simulink model "FCElectricPlant"  (R2025b)
settings: Solver=VariableStepAuto  StartTime=0.0  StopTime=2474  RelTol=1e-3
model workspace (MAT data in the model file):
  Bat.DischrgLmt_bpt = [0 0.35 0.7 1 1 1 1 1 1 1 1]
  Bat.ChrgLmt_bpt = [1 1 1 1 1 1 1 1 0.7 0.35 0]
  Bat.SOC_bpt = [0 0.1 0.2 0.3 0.4 0.5 0.6 0.7 0.8 0.9 1]
  Bat.BattDischrgMax = 110000
  Bat.BattChrgMax = -110000
  Bat.noLoadV = [201.6  201.6  201.6  201.6  201.6  201.6  201.6; 258.768  258.768  258.768  258.768  258.768  258.768  258.768; 264.96  264.96  264.96  264.96  264.96  264.96  264.96; 272.952  272.952  272.952  272.952  272.952  272.952  272.952; 286.128  286.128  286.128  286.128  286.128  286.128  286.128; 303.912  303.912  303.912  303.912  303.912  303.912  303.912]
  Bat.CapSOCBp = [0 0.2 0.4 0.6 0.8 1]
  Bat.BattTempBp = [243.1 253.1 263.1 273.1 283.1 298.1 313.1]
  Bat.CapLUTBp = [0 0.01 0.02 0.03 0.04 0.05 0.06 0.07 0.08 0.09 0.1 0.11 0.12 0.13 0.14 0.15 0.16 0.17 0.18 0.19 0.2 0.21 0.22 0.23 0.24 0.25 0.26 0.27 0.28 0.29 0.3 0.31 0.32 0.33 0.34 0.35 0.36 0.37 0.38 0.39 0.4 0.41 0.42 0.43 0.44 0.45 0.46 0.47 0.48 0.49 0.5 0.51 0.52 0.53 0.54 0.55 0.56 0.57 0.58 0.59 0.6 0.61 0.62 0.63 0.64 0.65 0.66 0.67 0.68 0.69 0.7 0.71 0.72 0.73 0.74 0.75 0.76 0.77 0.78 0.79 0.8 0.81 0.82 0.83 0.84 0.85 0.86 0.87 0.88 0.89 0.9 0.91 0.92 0.93 0.94 0.95 0.96 0.97 0.98 0.99 1]
  Bat.Em = [2.8 3.228 3.284 3.361 3.408 3.427 3.472 3.477 3.493 3.504 3.516 3.528 3.537 3.545 3.555 3.561 3.566 3.576 3.587 3.589 3.594 3.6 3.608 3.61 3.616 3.619 3.626 3.632 3.637 3.64 3.645 3.646 3.652 3.655 3.658 3.661 3.664 3.668 3.673 3.678 3.68 3.681 3.686 3.692 3.699 3.702 3.705 3.71 3.717 3.723 3.728 3.733 3.735 3.742 3.749 3.755 3.761 3.768 3.773 3.78 3.791 3.798 3.798 3.814 3.818 3.825 3.841 3.846 3.855 3.863 3.877 3.885 3.894 3.907 3.919 3.926 3.935 3.944 3.954 3.964 3.974 3.988 3.998 4.014 4.029 4.034 4.047 4.065 4.074 4.086 4.097 4.131 4.126 4.138 4.15 4.18 4.174 4.187 4.207 4.231 4.221]
  Bat.Ns = 72
  Bat.Np = 2
  Bat.BattChargeMax = 5.3
  Bat.BattCapInit = 3.18
  Bat.AH = [5.3 5.3 5.3 5.3 5.3 5.3 5.3]
  Bat.initSOC = 0.6
  Bat.RInt = [0.008846  0.006389  0.004364  0.002031  0.001443  0.0005603  0.001028; 0.009319  0.006554  0.004101  0.002563  0.001825  0.0007192  0.001338; 0.009027  0.005553  0.00406  0.002532  0.001795  0.0006887  0.001; 0.00847  0.005525  0.003452  0.00246  0.001778  0.0007557  0.001536; 0.01032  0.006043  0.003846  0.002716  0.001924  0.0007355  0.001546; 0.01314  0.007805  0.004517  0.003047  0.002234  0.001014  0.002789]
  Bat.R0 = [0.636912  0.460008  0.314208  0.146232  0.103896  0.0403416  0.074016; 0.670968  0.471888  0.295272  0.184536  0.1314  0.0517824  0.096336; 0.649944  0.399816  0.29232  0.182304  0.12924  0.0495864  0.072; 0.60984  0.3978  0.248544  0.17712  0.128016  0.0544104  0.110592; 0.74304  0.435096  0.276912  0.195552  0.138528  0.052956  0.111312; 0.94608  0.56196  0.325224  0.219384  0.160848  0.073008  0.200808]
  Bat.thermalMass = 500
  BattDCDC.Vout = 650
  BattDCDC.Plim = 60000
  BattDCDC.currMax = 9230.76923077
  BattDCDC.eff = 98
  BattDCDC.convLoss = 1
  BattDCDC.tc = 0.001
  BattDCDC.Vinit = 650
  BattDCDC.thermalMass = 500
  BattDCDC.Vdroop = 0
  BattDCDC.avgSwitchResistance = 0.001
  BattDCDC.diodeFwdVolt = 0.8
  BattDCDC.diodeOnResistance = 0.001
  BattDCDC.diodeOffConductance = 1e-05
  BattDCDC.inductance = 0.005
  BattDCDC.inductorSeriesResistance = 0
  BattDCDC.capacitance = 0.001
  BattDCDC.CapEffSeriesResistance = 10
  Brk.BrkPrsMax = 5000000
  Brk.mu_kinetic = 0.35
  Brk.mu_static = 0.45
  Brk.disk_abore = 0.05
  Brk.Rm = 0.15
  Brk.num_pads = 2
  Cond.Width = 60
  Cond.Height = 40
  Cond.Thickness = 2
  Cond.Area = 2400
  Cond.TubeDh = 0.25
  Cond.TubeArea = 0.0490873852123
  Cond.NTube = 256
  Cond.NPerRow = 8
  Cond.NRows = 32
  Cond.Spacing = 1
  Cond.TotFinArea = 30720
  Cpl.GearRatio = 1
  Cpl.Friction = 0.0001
  DH2 = 74
  DH2O = 25
  DO2 = 18
  DRVctrl.Ki = 1
  DRVctrl.Kp = 2
  Diff.Ndiff = 7.94
  Diff.Inertia = 0.5
  Driveshaft.inertia = 3
  Duct.Length = 5
  Duct.Width = 60
  Duct.Height = 40
  Duct.Area = 2400
  Duct.Dh = 48
  ElecThermal.ctrl.Kp = 0.1
  ElecThermal.ctrl.Ki = 0.1
  ElecThermal.TM1.mass = 2
  ElecThermal.TM1.sh = 910
  ElecThermal.Tank.volume = 0.001
  ElecThermal.Tank.area = 0.005
  ElecThermal.Tank.heightVector = [0.01 0.01]
  ElecThermal.Tank.areaVectorA1B1 = [0.001 0.001]
  ElecThermal.Tank.areaVectorA2B2 = [7.85398163397e-05 7.85398163397e-05]
  ElecThermal.MassFlowSource.area = 7.85398163397e-05
  ElecThermal.TL.bulkMod = 2.1791
  ElecThermal.TL.PressMin = 0.01
  ElecThermal.TL.PressMax = 50
  ElecThermal.TL.volumeFraction = 0.1
  ElecThermal.LR1.area = 3.92699081699e-05
  ElecThermal.LR1.areaAB = 7.85398163397e-05
  ElecThermal.LR1.cd = 0.7
  ElecThermal.LR1.RN = 12
  ElecThermal.P1.length = 1
  ElecThermal.P1.area = 7.85398163397e-05
  ElecThermal.P1.diam = 0.01
  ElecThermal.P1.elevGain = 0
  ElecThermal.P1.eqLength = 0.1
  ElecThermal.P1.rough = 1.5e-05
  ElecThermal.P1.lamDarcyFrac = 64
  ElecThermal.P1.lamUpp = 2000
  ElecThermal.P1.turbLow = 4000
  ElecThermal.P1.lamNu = 3.66
  ElecThermal.P2.length = 1
  ElecThermal.P2.area = 7.85398163397e-05
  ElecThermal.P2.diam = 0.01
  ElecThermal.P2.elevGain = 0
  ElecThermal.P2.eqLength = 0.1
  ElecThermal.P2.rough = 1.5e-05
  ElecThermal.P2.lamDarcyFrac = 64
  ElecThermal.P2.lamUpp = 2000
  ElecThermal.P2.turbLow = 4000
  ElecThermal.P2.lamNu = 3.66
  ElecThermal.P3.length = 1
  ElecThermal.P3.area = 7.85398163397e-05
  ElecThermal.P3.diam = 0.01
  ElecThermal.P3.elevGain = 0
  ElecThermal.P3.eqLength = 0.1
  ElecThermal.P3.rough = 1.5e-05
  ElecThermal.P3.lamDarcyFrac = 64
  ElecThermal.P3.lamUpp = 2000
  ElecThermal.P3.turbLow = 4000
  ElecThermal.P3.lamNu = 3.66
  FCDCDC.Vout = 650
  FCDCDC.Plim = 60000
  FCDCDC.Vdroop = 0
  FCDCDC.currMax = 9230.76923077
  FCDCDC.eff = 98
  FCDCDC.convLoss = 1
  FCDCDC.tc = 0.001
  FCDCDC.Vinit = 650
  FCDCDC.thermalMass = 500
  FCDCDC.conductance = 1e-08
  FCDCDC.inductance = 0.005
  FCDCDC.capacitance = 0.001
  FCDCDC.diodeFwdVolt = 0.8
  FCDCDC.diodeOnResistance = 0.001
  FCDCDC.diodeOffConductance = 1e-05
  FCDCDC.avgSwitchResistance = 0.001
  FCDCDC.inductorSeriesResistance = 0
  FCDCDC.CapEffSeriesResistance = 10
  FCctrl.maxPWR = 128000
  FCctrl.opLimit = 0.4
  FCctrl.minV = 200
  FCctrl.SOCtgt = 60
  FCctrl.tempTgt = 80
  FTP72.time = [0 0.00166966283167 0.00489789127635 0.00812611972102 0.01 0.0132225488916 0.0164450977832 0.0196676466748 0.02 0.0216617666259 0.024481578167 0.0273013897082 ... (181869 elements, 181869x1)]
  FTP72.SpdKph = [0 0 0 0 0 0 0 0 0 0 0 0 ... (181869 elements, 181869x1)]
  FTP75.time = [0 0.00166966283167 0.00489789127635 0.00812611972102 0.01 0.0132225488916 0.0164450977832 0.0196676466748 0.02 0.0216617666259 0.024481578167 0.0273013897082 ... (325038 elements, 325038x1)]
  FTP75.SpdKph = [0 0 0 0 0 0 0 0 0 0 0 0 ... (325038 elements, 325038x1)]
  FinArea = 2
  FinDensity = 4
  H2_D = 74
  H2_R = 4124.48151676
  H2_T = [-56.55 -50 -40 -30 -20 -10 -5 -4 -3 -2 -1 0 1 2 3 4 5 10 20 30 40 50 60 70 80 90 100 110 120 130 140 150 160 170 180 190 200 210 220 230 240 250 260 270 280 290 300 310 320 330 340 350]
  H2_h = [2783.66044046 2873.94181646 3012.62601981 3152.22537302 3292.62486344 3433.7213836 3504.50184296 3518.67512521 3532.85394544 3547.03822323 3561.22787913 3575.42283463 3589.62301216 3603.82833507 3618.03872764 3632.25411507 3646.47442344 3717.6472553 3860.32198735 4003.38288163 4146.77354613 4290.44463594 4434.35318484 4578.46197843 4722.73896833 4867.15672726 5011.69194457 5156.32496144 5301.03934494 5445.82149962 5590.66031514 5735.54684833 5880.47403768 6025.43644827 6170.43004499 6315.451992 6460.50047605 6605.57455183 6750.67400705 6895.79924544 7040.95118569 7186.13117474 7331.34091359 7476.58239436 7621.85784699 7767.16969457 7912.52051596 8057.91301484 8203.34999414 8348.83433523 8494.36898091 8639.95692183]
  H2_k = [142.834673487 146.602208511 152.236222043 157.732550942 163.09765294 168.338595937 170.914793442 171.426608923 171.937300227 172.446874689 172.955339635 173.462702375 173.968970204 174.474150403 174.978250232 175.481276935 175.983237736 178.477304495 183.389581256 188.206454189 192.934525091 197.580042888 202.148890501 206.646585109 211.078287131 215.448814629 219.762660868 224.024013436 228.236773895 232.404577248 236.530810786 240.618632037 244.670985681 248.690619345 252.680098287 256.641818973 260.578021603 264.490801638 268.382120403 272.253814814 276.107606319 279.945109096 283.767837587 287.577213413 291.374571729 295.161167068 298.938178719 302.706715675 306.467821201 310.222477041 313.971607306 317.716082068]
  H2_mu = [7.13280985169 7.28192581803 7.50683010986 7.72860158312 7.94743907375 8.16352107178 8.27057966039 8.29191522386 8.31322574339 8.33451136221 8.35577222214 8.37700846366 8.39822022586 8.41940764654 8.44057086215 8.46171000786 8.48282521754 8.58804682376 8.79676834159 9.00329345223 9.20773222364 9.41018554309 9.61074613692 9.80949945112 10.0065244149 10.2018941058 10.3956763308 10.5879341365 10.7787262582 10.9681075163 11.1561291684 11.3428392212 11.5282827091 11.7125019432 11.8955367341 12.0774245926 12.2582009096 12.4378991192 12.6165508457 12.7941860372 12.9708330866 13.1465189421 13.3212692073 13.4951082332 13.668059202 13.8401442043 14.0113843094 14.1817996299 14.3514093822 14.5202319407 14.6882848893 14.8555850676]
  HWFET.time = [0 0.00166966283167 0.00489789127635 0.00812611972102 0.01 0.0132225488916 0.0164450977832 0.0196676466748 0.02 0.0216617666259 0.024481578167 0.0273013897082 ... (82069 elements, 82069x1)]
  HWFET.SpdKph = [0 0 0 0 0 0 0 0 0 0 0 0 ... (82069 elements, 82069x1)]
  Mot.maxT = [335 335 335 335 335 269.767628541 215.814102833 179.845085694 154.152930595 134.88381427 119.896723796 107.907051416]
  Mot.w_eff_bp = [0 1000 2000 3000 3221 4000 5000 6000 7000 8000 9000 10000]
  Mot.Tc_Mot = 0.02
  Mot.T_eff_bp = [0 23.9285714286 47.8571428571 71.7857142857 95.7142857143 119.642857143 143.571428571 167.5 191.428571429 215.357142857 239.285714286 263.214285714 287.142857143 311.071428571 335]
  Mot.efficiency_table = [85  85  85  85  85  85  85  85  85  85  85  85  85  85  85; 85  85  85  85  85  85  85  85  85  85  85  85  85  85  85; 85  85  90  90  90  90  90  90  90  90  88  88  88  88  88; 85  85  92  92  92  92  92  92  92  92  92  90  90  90  90; 85  85  92  92  93  93  93  93  92  92  92  90  90  90  90; 85  85  93  94  94  94  94  94  94  94  94  94  94  94  94; 85  85  93  94  94  95  95  95  95  95  95  95  95  95  95; 85  85  93  94  94  95  95  95  95  95  95  95  95  95  95; 85  85  93  94  95  95  95  95  95  95  95  95  95  95  95; 85  85  93  94  95  95  95  95  95  95  95  95  95  95  95; 85  85  93  94  94  94  94  94  94  94  94  94  94  94  94; 85  85  90  92  93  93  93  93  93  93  93  93  93  93  93]
  Mot.supplyRes = 0
  Mot.inertia = 5e-06
  Mot.damping = 0
  Mot.thermalMass = 800
  Mot.winding.area = 250.2
  Mot.winding.thick = 1
  Mot.winding.cond = 401
  Mot.winding.mass = 5
  Mot.winding.sh = 385
  Mot.windingIron.area = 250
  Mot.windingIron.thick = 1
  Mot.windingIron.cond = 360
  Mot.windingIron.mass = 5
  Mot.windingIron.sh = 447
  Mot.ironStack.area = 4350
  Mot.ironStack.thick = 1
  Mot.ironStack.cond = 80.2
  Mot.ironStack.mass = 5
  Mot.ironStack.sh = 903
  N2_R = 296.802103844
  N2_T = [-56.55 -50 -40 -30 -20 -10 -5 -4 -3 -2 -1 0 1 2 3 4 5 10 20 30 40 50 60 70 80 90 100 110 120 130 140 150 160 170 180 190 200 210 220 230 240 250 260 270 280 290 300 310 320 330 340 350]
  N2_h = [224.312019476 231.141016529 241.564116975 251.984329606 262.402210767 272.818266127 278.025759131 279.06722248 280.10867517 281.150117667 282.191550441 283.232973957 284.274388686 285.315795097 286.357193658 287.39858484 288.439969116 293.646803475 304.060229226 314.473742204 324.887858161 335.303123494 345.720119003 356.139461811 366.561805672 376.987839946 387.41828743 397.853901301 408.295461341 418.743769659 429.199646055 439.663923199 450.137441735 460.621045431 471.115576471 481.621870952 492.140754651 502.673039103 513.219518026 523.780964099 534.358126107 544.951726469 555.562459109 566.190987693 576.837944198 587.503927793 598.18950402 608.895204248 619.621525378 630.368929765 641.137845362 651.928666026]
  N2_k = [19.6296532607 20.1533289725 20.9436243616 21.7231523445 22.4923063139 23.2514823267 23.6274403303 23.7023472872 23.7771601873 23.8518793809 23.9265052168 24.0010380424 24.0754782033 24.1498260439 24.2240819071 24.298246134 24.3723190645 24.7413260601 25.4726839899 26.1954347636 26.9098870601 27.616335804 28.3150627088 29.0063368423 29.6904152006 30.3675432786 31.0379556302 31.7018764132 32.3595199136 33.0110910506 33.656785857 34.2967919383 34.9312889073 35.560448797 36.1844364511 36.8034098926 37.4175206728 38.0269141997 38.6317300489 39.2321022558 39.8281595918 40.4200258249 41.0078199644 41.591656493 42.1716455849 42.7478933118 43.3205018374 43.8895696009 44.4551914905 45.0174590069 45.5764604183 46.1322809066]
  N2_mu = [13.7948920665 14.1367187352 14.6513506072 15.1575394446 15.6556177861 16.1459023391 16.3882166949 16.4364580271 16.4846261831 16.532721447 16.5807441017 16.6286944287 16.6765727079 16.7243792177 16.7721142355 16.8197780369 16.8673708962 17.1042805671 17.572933093 18.0349108462 18.4904598525 18.9398140034 19.38319572 19.820816593 20.2528779961 20.6795716689 21.1010802692 21.5175778944 21.9292305719 22.3361967211 22.7386275856 23.1366676392 23.5304549666 23.9201216192 24.3057939489 24.6875929203 25.0656344035 25.4400294479 25.8108845388 26.1783018382 26.5423794103 26.9032114332 27.260888397 27.615497291 27.9671217779 28.3158423592 28.6617365294 29.0048789219 29.3453414462 29.6831934166 30.0185016744 30.3513307024]
  NFin = 7680
  O2_D = 18
  O2_R = 259.836612623
  O2_T = [-56.55 -50 -40 -30 -20 -10 -5 -4 -3 -2 -1 0 1 2 3 4 5 10 20 30 40 50 60 70 80 90 100 110 120 130 140 150 160 170 180 190 200 210 220 230 240 250 260 270 280 290 300 310 320 330 340 350]
  O2_h = [196.314045635 202.302438243 211.445560194 220.590899229 229.740231593 238.895348953 243.475641264 244.39194743 245.308340402 246.224821996 247.14139403 248.05805832 248.974816681 249.891670932 250.808622886 251.725674358 252.642827164 257.230174605 266.413508633 275.609852765 284.820965751 294.048557918 303.294277513 312.559698674 321.846311316 331.155513044 340.488603076 349.846778084 359.231129801 368.642644209 378.082202098 387.550580811 397.04845695 406.576409877 416.134925825 425.724402468 435.345153816 444.997415319 454.681349062 464.397049 474.144546127 483.92381355 493.734771414 503.577291639 513.451202454 523.356292707 533.292315938 543.258994208 553.256021689 563.283068012 573.339781379 583.425791441]
  O2_k = [19.6661951881 20.2224765128 21.0645207725 21.898029696 22.7232456338 23.5404090718 23.9460452976 24.0269406553 24.1077592592 24.1885013406 24.2691671302 24.349756858 24.4302707537 24.5107090462 24.5910719638 24.6713597344 24.751572585 25.1515209479 25.9459275198 26.7331962712 27.5135401678 28.2871691203 29.0542797087 29.8150645641 30.569709483 31.3183935589 32.0612893462 32.7985630479 33.5303747184 34.2568784759 34.9782227188 35.6945503443 36.4059989645 37.1127011203 37.81478449 38.5123720922 39.2055824827 39.8945299436 40.5793246667 41.2600729279 41.9368772562 42.6098365938 43.2790464498 43.9445990477 44.6065834647 45.2650857659 45.9201891311 46.5719739769 47.2205180715 47.8658966458 48.5081824976 49.1474460917]
  O2_mu = [15.7665575307 16.1727626079 16.7849249434 17.3877315055 17.9815180942 18.5666055809 18.8559834763 18.9136105725 18.9711555252 19.0286186248 19.0860001607 19.1433004205 19.2005196907 19.2576582565 19.3147164018 19.3716944089 19.4285925592 19.7118952085 20.2726692662 20.8258892364 21.3718096795 21.9106736607 22.4427133237 22.9681504449 23.4871969667 24.0000555078 24.5069198497 25.0079753989 25.5033996256 25.9933624783 26.4780267762 26.9575485797 27.4320775393 27.9017572254 28.3667254388 28.8271145028 29.2830515394 29.7346587283 30.1820535522 30.625349027 31.0646539191 31.5000729504 31.9317069915 32.3596532436 32.7840054112 33.2048538637 33.6222857893 34.0363853397 34.4472337669 34.8549095533 35.2594885333 35.6610440103]
  PTctrl.RegenBrkCutOff = [0 1]
  PTctrl.RegenBrkSpd_bpt = [5 9]
  Pipe.Length = 750
  Pipe.Dh = 1.5
  Pipe.Area = 1.76714586764
  Pump.Speed = 4000
  Pump.Displacement = 40
  RH2 = 4124.48291466
  RH2O = 461.523115726
  RH_a = 0.6
  RH_c = 0.6
  RN2 = 296.802204439
  RO2 = 259.836700689
  RelayVariant = 1
  ScenarioIndex = 5
  Sig = Simulink.Signal
  Sig.Dimensions = -1
  Sig.DimensionsMode = 'auto'
  Sig.Complexity = 'auto'
  Sig.SampleTime = -1
  Sig.SamplingMode = 'auto'
  Sig.DataType = 'auto'
  SimEndTime = 2474
  T_cell = 80
  T_eff_bp = [0 20 40 60 80 100 120 140 160 180 200 220 240 260 280]
  T_env = 20
  T_ext = 30
  T_init = 303.15
  Tank.Volume = 10
  Tank.Area = 625
  Tank.WallArea = 2850
  Tire.Inertia = 0.2
  Tire.Rated_Vertical_Load = 3000
  Tire.Rated_Peak_Long_Force = 3500
  Tire.Slip_At_Peak_Force = 6
  Tire.Radius = 0.3
  Tvec = [-50 -40 -30 -20 -10 0 10 20 30 40 50 60 70 80 90 100 110 120 130 140 150 160 170 180 190 200 210 220 230 240 250 260 270 280 290 300 310 320 330 340 350]
  US06.time = [0 0.00166966283167 0.00489789127635 0.00812611972102 0.01 0.0132225488916 0.0164450977832 0.0196676466748 0.02 0.0216617666259 0.024481578167 0.0273013897082 ... (72955 elements, 72955x1)]
  US06.SpdKph = [0 0 0 0 0 0 0 0 0 0 0 0 ... (72955 elements, 72955x1)]
  UrbanCycle1.time = [0; 1; 2; 3; 4; 5; 6; 7; 8; 9; 10; 11; 12; 13; 14; 15; 16; 17; 18; 19; 20; 21; 22; 23; 24; 25; 26; 27; 28; 29; 30; 31; 32; 33; 34; 35; 36; 37; 38; 39; 40; 41; 42; 43; 44; 45; 46; 47; 48; 49; 50; 51; 52; 53; 54; 55; 56; 57; 58; 59; 60; 61; 62; 63; 64; 65; 66; 67; 68; 69; 70; 71; 72; 73; 74; 75; 76; 77; 78; 79; 80; 81; 82; 83; 84; 85; 86; 87; 88; 89; 90; 91; 92; 93; 94; 95; 96; 97; 98; 99; 100; 101; 102; 103; 104; 105; 106; 107; 108; 109; 110; 111; 112; 113; 114; 115; 116; 117; 118; 119; 120; 121; 122; 123; 124; 125; 126; 127; 128; 129; 130; 131; 132; 133; 134; 135; 136; 137; 138; 139; 140; 141; 142; 143; 144; 145; 146; 147; 148; 149; 150; 151; 152; 153; 154; 155; 156; 157; 158; 159; 160; 161; 162; 163; 164; 165; 166; 167; 168; 169; 170; 171; 172; 173; 174; 175; 176; 177; 178; 179; 180; 181; 182; 183; 184; 185; 186; 187; 188; 189; 190; 191; 192; 193; 194; 195]
  UrbanCycle1.SpdKph = [0; 0; 0; 0; 0; 0; 0; 0; 0; 0; 0; 0; 3.8; 7.5; 11.3; 15; 15; 15; 15; 15; 15; 15; 15; 15; 12; 9; 6; 3; 0; 0; 0; 0; 0; 0; 0; 0; 0; 0; 0; 0; 0; 0; 0; 0; 0; 0; 0; 0; 0; 0; 2.7; 5.3; 8; 10.7; 13.3; 16; 18.7; 21.3; 24; 26.7; 29.3; 32; 32; 32; 32; 32; 32; 32; 32; 32; 32; 32; 32; 32; 32; 32; 32; 32; 32; 32; 32; 32; 32; 32; 32; 32; 29.1; 26.2; 23.3; 20.4; 17.5; 14.5; 11.6; 8.7; 5.8; 2.9; 0; 0; 0; 0; 0; 0; 0; 0; 0; 0; 0; 0; 0; 0; 0; 0; 0; 0; 0; 0; 0; 0; 1.9; 3.8; 5.8; 7.7; 9.6; 11.5; 13.5; 15.4; 17.3; 19.2; 21.2; 23.4; 25; 26.9; 28.8; 30.8; 32.7; 34.6; 36.5; 38.5; 40.4; 42.3; 44.2; 46.2; 48.1; 50; 50; 50; 50; 50; 50; 50; 50; 50; 50; 50; 50; 50; 48.1; 46.2; 44.4; 42.5; 40.6; 38.8; 36.9; 35; 35; 35; 35; 35; 35; 35; 35; 35; 35; 35; 35; 35; 35; 32.1; 29.2; 26.2; 23.3; 20.4; 17.5; 14.6; 11.7; 8.7; 5.8; 2.9; 0; 0; 0; 0; 0; 0; 0; 0]
  UrbanCycle2.SpdKph = [0; 0; 0; 0; 0; 0; 0; 0; 0; 0; 0; 0; 0; 0; 0; 0; 0; 0; 0; 0; 0; 3; 6; 9; 12; 15; 15; 15; 17.2; 19.4; 21.7; 23.9; 26.1; 28.3; 30.6; 32.8; 35; 35; 35; 36.9; 38.8; 40.6; 42.5; 44.4; 46.3; 48.1; 50; 50; 50; 51.5; 53.1; 54.6; 56.2; 57.7; 59.2; 60.8; 62.3; 63.8; 65.4; 66.9; 68.5; 70; 70; 70; 70; 70; 70; 70; 70; 70; 70; 70; 70; 70; 70; 70; 70; 70; 70; 70; 70; 70; 70; 70; 70; 70; 70; 70; 70; 70; 70; 70; 70; 70; 70; 70; 70; 70; 70; 70; 70; 70; 70; 70; 70; 70; 70; 70; 70; 70; 70; 70; 67.5; 65; 62.5; 60; 57.5; 55; 52.5; 50; 50; 50; 50; 50; 50; 50; 50; 50; 50; 50; 50; 50; 50; 50; 50; 50; 50; 50; 50; 50; 50; 50; 50; 50; 50; 50; 50; 50; 50; 50; 50; 50; 50; 50; 50; 50; 50; 50; 50; 50; 50; 50; 50; 50; 50; 50; 50; 50; 50; 50; 50; 50; 50; 50; 50; 50; 50; 50; 50; 50; 50; 50; 50; 50; 50; 50; 50; 50; 50; 51.5; 53.1; 54.6; 56.2; 57.7; 59.2; 60.8; 62.3; 63.8; 65.4; 66.9; 68.5; 70; 70; 70; 70; 70; 70; 70; 70; 70; 70; 70; 70; 70; 70; 70; 70; 70; 70; 70; 70; 70; 70; 70; 70; 70; 70; 70; 70; 70; 70; 70; 70; 70; 70; 70; 70; 70; 70; 70; 70; 70; 70; 70; 70; 70; 70; 70; 70; 70; 70; 70; 70.9; 71.7; 72.6; 73.4; 74.3; 75.1; 76; 76.9; 77.7; 78.6; 79.4; 80.3; 81.1; 82; 82.9; 83.7; 84.6; 85.4; 86.3; 87.1; 88; 88.9; 89.7; 90.6; 91.4; 92.3; 93.1; 94; 94.9; 95.7; 96.6; 97.4; 98.3; 99.1; 100; 100; 100; 100; 100; 100; 100; 100; 100; 100; 100; 100; 100; 100; 100; 100; 100; 100; 100; 100; 100; 100; 100; 100; 100; 100; 100; 100; 100; 100; 100; 101; 102; 103; 104; 105; 106; 107; 108; 109; 110; 111; 112; 113; 114; 115; 116; 117; 118; 119; 120; 120; 120; 120; 120; 120; 120; 120; 120; 120; 120; 117.5; 115; 112.5; 110; 107.5; 105; 102.5; 100; 97.5; 95; 92.5; 90; 87.5; 85; 82.5; 80; 76.3; 72.5; 68.8; 65; 61.3; 57.5; 53.8; 50; 45; 40; 35; 30; 25; 20; 15; 10; 5; 0; 0; 0; 0; 0; 0; 0; 0; 0; 0; 0; 0; 0; 0; 0; 0; 0; 0; 0; 0; 0]
  UrbanCycle2.time = [0; 1; 2; 3; 4; 5; 6; 7; 8; 9; 10; 11; 12; 13; 14; 15; 16; 17; 18; 19; 20; 21; 22; 23; 24; 25; 26; 27; 28; 29; 30; 31; 32; 33; 34; 35; 36; 37; 38; 39; 40; 41; 42; 43; 44; 45; 46; 47; 48; 49; 50; 51; 52; 53; 54; 55; 56; 57; 58; 59; 60; 61; 62; 63; 64; 65; 66; 67; 68; 69; 70; 71; 72; 73; 74; 75; 76; 77; 78; 79; 80; 81; 82; 83; 84; 85; 86; 87; 88; 89; 90; 91; 92; 93; 94; 95; 96; 97; 98; 99; 100; 101; 102; 103; 104; 105; 106; 107; 108; 109; 110; 111; 112; 113; 114; 115; 116; 117; 118; 119; 120; 121; 122; 123; 124; 125; 126; 127; 128; 129; 130; 131; 132; 133; 134; 135; 136; 137; 138; 139; 140; 141; 142; 143; 144; 145; 146; 147; 148; 149; 150; 151; 152; 153; 154; 155; 156; 157; 158; 159; 160; 161; 162; 163; 164; 165; 166; 167; 168; 169; 170; 171; 172; 173; 174; 175; 176; 177; 178; 179; 180; 181; 182; 183; 184; 185; 186; 187; 188; 189; 190; 191; 192; 193; 194; 195; 196; 197; 198; 199; 200; 201; 202; 203; 204; 205; 206; 207; 208; 209; 210; 211; 212; 213; 214; 215; 216; 217; 218; 219; 220; 221; 222; 223; 224; 225; 226; 227; 228; 229; 230; 231; 232; 233; 234; 235; 236; 237; 238; 239; 240; 241; 242; 243; 244; 245; 246; 247; 248; 249; 250; 251; 252; 253; 254; 255; 256; 257; 258; 259; 260; 261; 262; 263; 264; 265; 266; 267; 268; 269; 270; 271; 272; 273; 274; 275; 276; 277; 278; 279; 280; 281; 282; 283; 284; 285; 286; 287; 288; 289; 290; 291; 292; 293; 294; 295; 296; 297; 298; 299; 300; 301; 302; 303; 304; 305; 306; 307; 308; 309; 310; 311; 312; 313; 314; 315; 316; 317; 318; 319; 320; 321; 322; 323; 324; 325; 326; 327; 328; 329; 330; 331; 332; 333; 334; 335; 336; 337; 338; 339; 340; 341; 342; 343; 344; 345; 346; 347; 348; 349; 350; 351; 352; 353; 354; 355; 356; 357; 358; 359; 360; 361; 362; 363; 364; 365; 366; 367; 368; 369; 370; 371; 372; 373; 374; 375; 376; 377; 378; 379; 380; 381; 382; 383; 384; 385; 386; 387; 388; 389; 390; 391; 392; 393; 394; 395; 396; 397; 398; 399; 400]
  UrbanCycle3.time = [0; 1; 2; 3; 4; 5; 6; 7; 8; 9; 10; 11; 12; 13; 14; 15; 16; 17; 18; 19; 20; 21; 22; 23; 24; 25; 26; 27; 28; 29; 30; 31; 32; 33; 34; 35; 36; 37; 38; 39; 40; 41; 42; 43; 44; 45; 46; 47; 48; 49; 50; 51; 52; 53; 54; 55; 56; 57; 58; 59; 60; 61; 62; 63; 64; 65; 66; 67; 68; 69; 70; 71; 72; 73; 74; 75; 76; 77; 78; 79; 80; 81; 82; 83; 84; 85; 86; 87; 88; 89; 90; 91; 92; 93; 94; 95; 96; 97; 98; 99; 100; 101; 102; 103; 104; 105; 106; 107; 108; 109; 110; 111; 112; 113; 114; 115; 116; 117; 118; 119; 120; 121; 122; 123; 124; 125; 126; 127; 128; 129; 130; 131; 132; 133; 134; 135; 136; 137; 138; 139; 140; 141; 142; 143; 144; 145; 146; 147; 148; 149; 150; 151; 152; 153; 154; 155; 156; 157; 158; 159; 160; 161; 162; 163; 164; 165; 166; 167; 168; 169; 170; 171; 172; 173; 174; 175; 176; 177; 178; 179; 180; 181; 182; 183; 184; 185; 186; 187; 188; 189; 190; 191; 192; 193; 194; 195; 196; 197; 198; 199; 200; 201; 202; 203; 204; 205; 206; 207; 208; 209; 210; 211; 212; 213; 214; 215; 216; 217; 218; 219; 220; 221; 222; 223; 224; 225; 226; 227; 228; 229; 230; 231; 232; 233; 234; 235; 236; 237; 238; 239; 240; 241; 242; 243; 244; 245; 246; 247; 248; 249; 250; 251; 252; 253; 254; 255; 256; 257; 258; 259; 260; 261; 262; 263; 264; 265; 266; 267; 268; 269; 270; 271; 272; 273; 274; 275; 276; 277; 278; 279; 280; 281; 282; 283; 284; 285; 286; 287; 288; 289; 290; 291; 292; 293; 294; 295; 296; 297; 298; 299; 300; 301; 302; 303; 304; 305; 306; 307; 308; 309; 310; 311; 312; 313; 314; 315; 316; 317; 318; 319; 320; 321; 322; 323; 324; 325; 326; 327; 328; 329; 330; 331; 332; 333; 334; 335; 336; 337; 338; 339; 340; 341; 342; 343; 344; 345; 346; 347; 348; 349; 350; 351; 352; 353; 354; 355; 356; 357; 358; 359; 360; 361; 362; 363; 364; 365; 366; 367; 368; 369; 370; 371; 372; 373; 374; 375; 376; 377; 378; 379; 380; 381; 382; 383; 384; 385; 386; 387; 388; 389; 390; 391; 392; 393; 394; 395; 396; 397; 398; 399; 400]
  UrbanCycle3.SpdKph = [0; 0; 0; 0; 0; 0; 0; 0; 0; 0; 0; 0; 0; 0; 0; 0; 0; 0; 0; 0; 0; 3; 6; 9; 12; 15; 15; 15; 17.2; 19.4; 21.7; 23.9; 26.1; 28.3; 30.6; 32.8; 35; 35; 35; 36.9; 38.8; 40.6; 42.5; 44.4; 46.3; 48.1; 50; 50; 50; 51.5; 53.1; 54.6; 56.2; 57.7; 59.2; 60.8; 62.3; 63.8; 65.4; 66.9; 68.5; 70; 70; 70; 70; 70; 70; 70; 70; 70; 70; 70; 70; 70; 70; 70; 70; 70; 70; 70; 70; 70; 70; 70; 70; 70; 70; 70; 70; 70; 70; 70; 70; 70; 70; 70; 70; 70; 70; 70; 70; 70; 70; 70; 70; 70; 70; 70; 70; 70; 70; 70; 67.5; 65; 62.5; 60; 57.5; 55; 52.5; 50; 50; 50; 50; 50; 50; 50; 50; 50; 50; 50; 50; 50; 50; 50; 50; 50; 50; 50; 50; 50; 50; 50; 50; 50; 50; 50; 50; 50; 50; 50; 50; 50; 50; 50; 50; 50; 50; 50; 50; 50; 50; 50; 50; 50; 50; 50; 50; 50; 50; 50; 50; 50; 50; 50; 50; 50; 50; 50; 50; 50; 50; 50; 50; 50; 50; 50; 50; 50; 50; 51.5; 53.1; 54.6; 56.2; 57.7; 59.2; 60.8; 62.3; 63.8; 65.4; 66.9; 68.5; 70; 70; 70; 70; 70; 70; 70; 70; 70; 70; 70; 70; 70; 70; 70; 70; 70; 70; 70; 70; 70; 70; 70; 70; 70; 70; 70; 70; 70; 70; 70; 70; 70; 70; 70; 70; 70; 70; 70; 70; 70; 70; 70; 70; 70; 70; 70; 70; 70; 70; 70; 70.8; 71.7; 72.5; 73.3; 74.2; 75; 75.8; 76.7; 77.5; 78.3; 79.2; 80; 80.8; 81.7; 82.5; 83.3; 84.2; 85; 85.8; 86.7; 87.5; 88.3; 89.2; 90; 90; 90; 90; 90; 90; 90; 90; 90; 90; 90; 90; 90; 90; 90; 90; 90; 90; 90; 90; 90; 90; 90; 90; 90; 90; 90; 90; 90; 90; 90; 90; 90; 90; 90; 90; 90; 90; 90; 90; 90; 90; 90; 90; 90; 90; 90; 90; 90; 90; 90; 90; 90; 90; 90; 90; 90; 90; 90; 90; 90; 90; 90; 90; 90; 90; 90; 90; 90; 90; 90; 90; 90; 90; 90; 90; 90; 90; 90; 90; 90; 90; 90; 90; 87.5; 85; 82.5; 80; 76.3; 72.5; 68.8; 65; 61.3; 57.5; 53.8; 50; 45; 40; 35; 30; 25; 20; 15; 10; 5; 0; 0; 0; 0; 0; 0; 0; 0; 0; 0; 0; 0; 0; 0; 0; 0; 0; 0; 0; 0; 0]
  UrbanCycle4.time = [0 1 2 3 4 5 6 7 8 9 10 11 ... (507 elements, 507x1)]
  UrbanCycle4.SpdKph = [0 0 0 0 0 0 0 0 0 0 0 0 ... (507 elements, 507x1)]
  UrbanCycle5.time = [0 1 2 3 4 5 6 7 8 9 10 11 ... (661 elements, 661x1)]
  UrbanCycle5.SpdKph = [0 0 0 0 0 0 0 0 0 0 0 0 ... (661 elements, 661x1)]
  Vehicle.Mass = 1800
  Vehicle.Distance_CG_FrontAxle = 1.35
  Vehicle.Distance_CG_RearAxle = 1.35
  Vehicle.Distance_CG_Ground = 0.5
  Vehicle.Frontal_Area = 2.16
  Vehicle.Aero_Drag_Coeff = 0.26
  WOT.time = [0 0.00166966283167 0.00489789127635 0.00812611972102 0.01 0.0132225488916 0.0164450977832 0.0196676466748 0.02 0.0216617666259 0.024481578167 0.0273013897082 ... (6347 elements, 6347x1)]
  WOT.SpdKph = [0 0 0 0 0 0 0 0 0 0 0 0 ... (6347 elements, 6347x1)]
  anode_tube_D = 0.01
  cathode_tube_D = 0.05
  comp_mdot_corr_TLU = [0  0.2  0.4; 0  0.15  0.3; 0  0.1  0.2; 0  0.05  0.1; 0  0  0]
  comp_p_ratio_TLU = [1; 1.25; 1.5; 1.75; 2]
  comp_rpm_TLU = [0 1800 3600]
  coolant_num_layers = 20
  coolant_num_passes = 12
  coolant_tube_D = 0.05
  coolant_w_channels = 1
  drive_cycle_power = [0 0 0 0 0 0 0 0 0 0 0 0 ... (1050 elements, 1050x1)]
  drive_cycle_time = [0 3.15544362088e-30 0.0046730644306 0.0046730644306 0.0229169980413 0.0229169980413 0.0411609316521 0.0594048652628 0.0958927324843 0.168868466927 0.308339923682 0.308339923682 ... (1050 elements, 1050x1)]
  efficiency_table = [85  85  85  85  85  85  85  85  85  85  85  85  85  85  85; 85  85  85  85  85  85  85  85  85  85  85  85  85  85  85; 85  85  90  90  90  90  90  90  90  90  88  88  88  88  88; 85  85  92  92  92  92  92  92  92  92  92  90  90  90  90; 85  85  92  92  93  93  93  93  92  92  92  90  90  90  90; 85  85  93  94  94  94  94  94  94  94  94  94  94  94  94; 85  85  93  94  94  95  95  95  95  95  95  95  95  95  95; 85  85  93  94  94  95  95  95  95  95  95  95  95  95  95; 85  85  93  94  95  95  95  95  95  95  95  95  95  95  95; 85  85  93  94  95  95  95  95  95  95  95  95  95  95  95; 85  85  93  94  94  94  94  94  94  94  94  94  94  94  94; 85  85  90  92  93  93  93  93  93  93  93  93  93  93  93]
  env_RH = 0.5
  env_T = 20
  env_p = 0.101325
  env_yO2 = 0.21
  f_fc_auxpower = [551.873653203 546.0853282 528.48462663 513.173595038 503.302975177 502.753456089 515.021163214 542.265022773 584.751680012 640.816461254 707.312051903 780.384247238 ... (869 elements, 79x11)]
  f_fc_currcmd_bpt = [0.209765 5.20060185897 10.1914387179 15.1822755769 20.1731124359 25.1639492949 30.1547861538 35.1456230128 40.1364598718 45.1272967308 50.1181335897 55.1089704487 60.0998073077 65.0906441667 70.0814810256 75.0723178846 80.0631547436 85.0539916026 90.0448284615 95.0356653205 100.026502179 105.017339038 110.008175897 114.999012756 119.989849615 124.980686474 129.971523333 134.962360192 139.953197051 144.94403391 149.934870769 154.925707628 159.916544487 164.907381346 169.898218205 174.889055064 179.879891923 184.870728782 189.861565641 194.8524025 199.843239359 204.834076218 209.824913077 214.815749936 219.806586795 224.797423654 229.788260513 234.779097372 239.769934231 244.76077109 249.751607949 254.742444808 259.733281667 264.724118526 269.714955385 274.705792244 279.696629103 284.687465962 289.678302821 294.669139679 299.659976538 304.650813397 309.641650256 314.632487115 319.623323974 324.614160833 329.604997692 334.595834551 339.58667141 344.577508269 349.568345128 354.559181987 359.550018846 364.540855705 369.531692564 374.522529423 379.513366282 384.504203141 389.49504]
  f_fc_h2flow = [8.71593619412e-08 2.11208831613e-05 4.21802637945e-05 6.3315607286e-05 8.44733435522e-05 0.000105614873893 0.000126714989157 0.000147760022647 0.000168745833381 0.000189675717181 0.000210558338983 0.000231405772833 ... (869 elements, 79x11)]
  f_fc_heatflow = [-113.508553924 315.682858012 683.83093304 1077.33211881 1492.74924564 1928.28255982 2383.1090309 2856.86201514 3349.28475785 3860.05320307 4388.73420272 4934.82889994 ... (869 elements, 79x11)]
  f_fc_tmpcmd_bpt = [50 55 60 65 70 75 80 85 90 95 100]
  f_fc_voltage = [454.992615106 449.926167951 444.44198715 439.413829244 434.829610174 430.668984057 426.90491616 423.505302786 420.434569606 417.655187333 415.129053553 412.818701247 ... (869 elements, 79x11)]
  hH2 = [2873941.81645 3012626.01981 3152225.37301 3292624.86344 3433721.38359 3575422.83463 3717647.2553 3860321.98734 4003382.88163 4146773.54613 4290444.63593 4434353.18483 4578461.97843 4722738.96833 4867156.72726 5011691.94456 5156324.96143 5301039.34494 5445821.49962 5590660.31514 5735546.84833 5880474.03768 6025436.44826 6170430.04499 6315451.99199 6460500.47604 6605574.55182 6750674.00704 6895799.24543 7040951.18568 7186131.17473 7331340.91359 7476582.39435 7621857.84698 7767169.69456 7912520.51596 8057913.01483 8203349.99414 8348834.33523 8494368.98091 8639956.92183]
  hH2O = [2407979.18389 2426599.35505 2445219.52621 2463839.69737 2482459.86853 2501080.03969 2520041.36444 2538661.5356 2557304.93352 2575974.09714 2594671.5511 2613399.77792 2632161.19415 2650958.13077 2669792.81764 2688667.37205 2707583.79088 2726543.94613 2745549.58335 2764602.32251 2783703.66092 2802854.97781 2822057.54008 2841312.50904 2860620.94768 2879983.8283 2899402.0402 2918876.39739 2938407.64597 2957996.47114 2977643.50384 2997349.32672 3017114.47952 3036939.46377 3056824.74662 3076770.76378 3096777.92136 3116846.59619 3136977.13407 3157169.84449 3177424.99]
  hN2 = [231141.016491 241564.116943 251984.329578 262402.210743 272818.266107 283232.973942 293646.803464 304060.22922 314473.742203 324887.858166 335303.123505 345720.119022 356139.461838 366561.80571 376987.839995 387418.287492 397853.901378 408295.461435 418743.769771 429199.646188 439663.923356 450137.441917 460621.045642 471115.576713 481621.871228 492140.754963 502673.039455 513219.518421 523780.964538 534358.126595 544951.727008 555562.459702 566190.988344 576837.944909 587503.928567 598189.50486 608895.205157 619621.526358 630368.93082 641137.846494 651928.667237]
  hO2 = [202302.438244 211445.560195 220590.89923 229740.231594 238895.348953 248058.05832 257230.174606 266413.508634 275609.852766 284820.965752 294048.557919 303294.277514 312559.698674 321846.311316 331155.513045 340488.603077 349846.778085 359231.129802 368642.644209 378082.202099 387550.580812 397048.456951 406576.409878 416134.925826 425724.402468 435345.153817 444997.41532 454681.349063 464397.049001 474144.546128 483923.813551 493734.771415 503577.291639 513451.202454 523356.292708 533292.315939 543258.994209 553256.02169 563283.068013 573339.78138 583425.791442]
  hvH2O = [2837864.0802 2838666.81899 2838713.54467 2838009.25742 2836579.406 2834477.18894 2477187.06302 2453519.25942 2429811.22988 2405977.28679 2381947.12654 2357654.5203 2333031.20801 2308003.52809 2282490.62772 2256403.72153 2229646.15315 2202114.07337 2173697.48076 2144281.28269 2113746.00965 2081967.88341 2048818.0713 2014161.09963 1977852.49331 1939735.72817 1899638.5239 1857368.38273 1812707.10332 1765403.78805 1715165.61416 1661645.2634 1604423.22494 1542982.06457 1476667.90089 1404630.83498 1325728.75296 1238362.12284 1140162.8135 1027316.58329 892746.804216]
  kH2 = [0.14660211438 0.15223611697 0.157732436203 0.163097529696 0.168338465237 0.173462565161 0.178477161614 0.183389433463 0.188206302164 0.192934369439 0.197579884152 0.202148729169 0.206646421619 0.211078121877 0.215448647967 0.21976249312 0.224023844894 0.228236604824 0.232404407893 0.236530641368 0.240618462761 0.244670816735 0.248690450904 0.252679930513 0.256641652017 0.260577855606 0.264490636733 0.268381956715 0.272253652461 0.276107445413 0.279944949744 0.283767679891 0.287577057471 0.291374417634 0.295161014911 0.298938028586 0.302706567652 0.30646767537 0.310222333482 0.313971466098 0.317715943287]
  kH2O = [0.0133993325489 0.0140727292017 0.0147461258545 0.0154195225073 0.0160929191601 0.0167663158129 0.017416450238 0.0180898468908 0.0187835182831 0.019496836926 0.0202291830642 0.0209799564979 0.0217485824984 0.022534514185 0.0233372328149 0.0241562468853 0.0249910906022 0.0258413220573 0.0267065213239 0.027586288594 0.0284802424289 0.0293880181591 0.0303092664468 0.0312436520137 0.0321908525251 0.0331505576189 0.0341224680656 0.0351062950429 0.0361017595124 0.0371085916839 0.0381265305554 0.039155323521 0.0401947260356 0.0412445013363 0.0423044202141 0.0433742608421 0.0444538086676 0.0455428563902 0.046641204073 0.047748659475 0.048865038743]
  kN2 = [0.0201533289599 0.0209436243479 0.0217231523299 0.0224923062983 0.0232514823103 0.0240010380251 0.0247413260421 0.0254726839711 0.026195434744 0.0269098870397 0.0276163357829 0.028315062687 0.0290063368199 0.0296904151774 0.0303675432547 0.0310379556057 0.031701876388 0.0323595198879 0.0330110910242 0.03365678583 0.0342967919107 0.0349312888791 0.0355604487682 0.0361844364218 0.0368034098627 0.0374175206423 0.0380269141687 0.0386317300173 0.0392321022236 0.0398281595592 0.0404200257917 0.0410078199307 0.0415916564588 0.0421716455502 0.0427478932766 0.0433205018017 0.0438895695647 0.0444551914538 0.0450174589697 0.0455764603806 0.0461322808684]
  kO2 = [0.0202224764979 0.0210645207571 0.0218980296803 0.0227232456176 0.0235404090551 0.0243497568408 0.0251515209302 0.0259459275017 0.0267331962527 0.0275135401488 0.0282871691008 0.0290542796888 0.0298150645436 0.0305697094621 0.0313183935376 0.0320612893244 0.0327985630256 0.0335303746957 0.0342568784527 0.0349782226953 0.0356945503203 0.03640599894 0.0371127010954 0.0378147844647 0.0385123720666 0.0392055824566 0.0398945299172 0.0405793246398 0.0412600729007 0.0419368772286 0.0426098365657 0.0432790464214 0.0439445990189 0.0446065834356 0.0452650857363 0.0459201891012 0.0465719739465 0.0472205180409 0.0478658966148 0.0485081824662 0.04914744606]
  muH2 = [7.28192631884e-06 7.50683062629e-06 7.72860211493e-06 7.94743962074e-06 8.16352163375e-06 8.37700904042e-06 8.58804741514e-06 8.79676894741e-06 9.00329407235e-06 9.20773285791e-06 9.41018619135e-06 9.61074679906e-06 9.809500127e-06 1.00065251044e-05 1.02018948088e-05 1.03956770472e-05 1.05879348662e-05 1.0778727001e-05 1.09681082723e-05 1.11561299374e-05 1.1342840003e-05 1.15282835037e-05 1.17125027505e-05 1.18955375541e-05 1.20774254252e-05 1.22582017546e-05 1.24378999766e-05 1.26165517154e-05 1.27941869192e-05 1.29708339808e-05 1.31465198485e-05 1.33212701257e-05 1.34951091636e-05 1.36680601444e-05 1.38401451585e-05 1.40113852754e-05 1.41818006077e-05 1.43514103717e-05 1.45202329419e-05 1.4688285902e-05 1.48555860919e-05]
  muH2O = [7.40754821278e-06 7.71570492949e-06 8.0238616462e-06 8.33201836291e-06 8.64017507962e-06 8.94833179633e-06 9.24231634895e-06 9.55047306566e-06 9.87031914628e-06 1.02003383346e-05 1.05392900589e-05 1.08861429187e-05 1.12400271296e-05 1.16001998721e-05 1.19660196026e-05 1.23369267066e-05 1.27124287135e-05 1.30920888432e-05 1.34755170214e-05 1.38623627459e-05 1.42523093607e-05 1.46450694092e-05 1.50403808272e-05 1.54380037934e-05 1.5837718101e-05 1.6239320946e-05 1.66426250507e-05 1.70474570612e-05 1.74536561678e-05 1.78610729109e-05 1.82695681407e-05 1.86790121055e-05 1.90892836493e-05 1.9500269501e-05 1.99118636434e-05 2.03239667489e-05 2.07364856747e-05 2.11493330075e-05 2.15624266528e-05 2.19756894601e-05 2.23890488821e-05]
  muN2 = [1.41367187228e-05 1.46513505944e-05 1.51575394313e-05 1.56556177724e-05 1.6145902325e-05 1.66286944141e-05 1.71042805521e-05 1.75729330776e-05 1.80349108304e-05 1.84904598363e-05 1.89398139868e-05 1.9383195703e-05 1.98208165756e-05 2.02528779784e-05 2.06795716508e-05 2.11010802507e-05 2.15175778755e-05 2.19292305527e-05 2.23361967016e-05 2.27386275656e-05 2.31366676189e-05 2.3530454946e-05 2.39201215982e-05 2.43057939276e-05 2.46875928987e-05 2.50656343816e-05 2.54400294256e-05 2.58108845161e-05 2.61783018152e-05 2.6542379387e-05 2.69032114096e-05 2.72608883731e-05 2.76154972668e-05 2.79671217534e-05 2.83158423343e-05 2.86617365042e-05 2.90048788965e-05 2.93453414205e-05 2.96831933906e-05 3.00185016481e-05 3.03513306758e-05]
  muO2 = [1.6172762594e-05 1.67849249289e-05 1.73877314906e-05 1.79815180788e-05 1.8566605565e-05 1.9143300404e-05 1.97118951916e-05 2.02726692488e-05 2.08258892185e-05 2.13718096611e-05 2.19106736419e-05 2.24427133044e-05 2.29681504252e-05 2.34871969465e-05 2.40000554872e-05 2.45069198286e-05 2.50079753774e-05 2.55033996037e-05 2.59933624559e-05 2.64780267534e-05 2.69575485565e-05 2.74320775157e-05 2.79017572014e-05 2.83667254144e-05 2.88271144781e-05 2.92830515142e-05 2.97346587027e-05 3.01820535262e-05 3.06253490007e-05 3.10646538924e-05 3.15000729233e-05 3.1931706964e-05 3.23596532158e-05 3.2784005383e-05 3.32048538352e-05 3.36222857604e-05 3.40363853104e-05 3.44472337373e-05 3.48549095233e-05 3.5259488503e-05 3.56610439797e-05]
  pH2O = [0.0039376926592 0.0128411282011 0.0380050105363 0.103238678713 0.259872929049 0.611151401419 1.22819893069 2.33931818334 4.24697083683 7.38493807375 12.3519458375 19.9464343078 31.2009300265 47.4144740302 70.1817658151 101.41799666 143.378712949 198.67442048 270.279976785 361.5390994 476.16453797 618.234621425 792.187006981 1002.81053608 1255.23615516 1554.92790047 1907.67499353 2319.5861702 2797.08749693 3346.92514427 3976.17493065 4692.2609923 5502.98678301 6416.58290953 7441.77834442 8587.90494083 9865.05121118 11284.2929275 12858.0516 14600.6773719 16529.415139]
  p_a = 0.101325
  p_c = 0.101325
  p_sat = 0.0474144740302
  p_sat_c = 0.0474144740302
  p_sat_e = 0.00233931818334
  radiator_H = 0.5
  radiator_L = 1
  radiator_N_fins = 12000
  radiator_N_tubes = 25
  radiator_W = 0.025
  radiator_air_area_fins = 11.5625
  radiator_air_area_primary = 1.223125
  radiator_cp = 910
  radiator_eta_fin = 0.7
  radiator_fin_spacing = 0.002
  radiator_gap_H = 0.0192708333333
  radiator_rho = 2700
  radiator_t_wall = 0.0001
  radiator_tube_H = 0.0015
  radiator_tube_Leq = 2.5
  stack_D_gdl = 0.07
  stack_alpha = 0.6
  stack_area = 280
  stack_iL = 1.4
  stack_io = 0.0001
  stack_mea_cp = 870
  stack_mea_rho = 1800
  stack_membrane_MW = 1.1
  stack_membrane_rho = 2000
  stack_num_cells = 400
  stack_num_channels = 8
  stack_t_gdl = 250
  stack_t_membrane = 125
  stack_w_channels = 1
  tank_V = 120
  tank_p = 70
  tank_yH2 = 0.9997
  y_H2O_a = 0.280766685597
  y_H2O_c = 0.0138523652603
  y_H2_a = 0.719233314403
  y_N2_a = 0
  y_N2_c = 0.77614763474
  y_O2_c = 0.21
libraries: fl_lib x91, nesl_utility x43, autolibpowerinfoutils x9, SimscapeFluids_lib x5, ee_lib x3, slpidlib x2, batteryecm_lib x1, simulink_extras x1, simulink x1
(part 1 of 4)
settings Model: DataDictionary=FCElectricPlant.sldd  ModifiedByFormat=The MathWorks, Inc.  SimulationMode=accelerator  Creator=The MathWorks, Inc.  LastModifiedBy=The MathWorks, Inc.
settings SolverCC: ZeroCrossAlgorithm=Adaptive  AlgebraicLoopSolver=TrustRegion  AutoInsertRateTranBlk=on  DecoupledContinuousIntegration=on  MinimalZcImpactIntegration=on  MaxZcPerStep=1.0
settings DataIOCC: SaveOutput=off  DSMLogging=off  SaveTime=off  ReturnWorkspaceOutputs=off
settings OptimizationCC: ReuseModelBlockBuffer=off  EfficientMapNaN2IntZero=off
settings DebuggingCC: ArtificialAlgebraicLoopMsg=none  MaskedZcDiagnostic=none  IgnoredZcDiagnostic=none  UnconnectedInputMsg=warning  UnconnectedOutputMsg=warning  UnconnectedLineMsg=warning  SubsystemReferenceDiagnosticForUnitTest=warning  SymbolicDimsDataTypeCodeGenerationDiagnostic=none  ArithmeticOperatorsInVariantConditions=warning
settings HardwareCC: TargetIntDivRoundTo=Zero  TargetEndianess=LittleEndian  TargetHWDeviceType=Custom Processor->Custom Processor  ProdEqTarget=off
settings ModelReferenceCC: UpdateModelReferenceTargets=IfOutOfDate  EnableRefExpFcnMdlSchedulingChecks=on  PropagateSignalLabelsOutOfModel=off
settings SFSimCC: CustomCodeUndefinedFunction=UseInterfaceOnly
settings RTWCC: GPUComputeCapability=3.5  DLArmComputeVersion=19.05
settings CodeAppCC: MaxIdLength=128.0
settings SimscapeCC: SimscapeLogSimulationStatistics=on  SimscapeLogLimitData=off  SimscapeLogDataHistory=10000.0

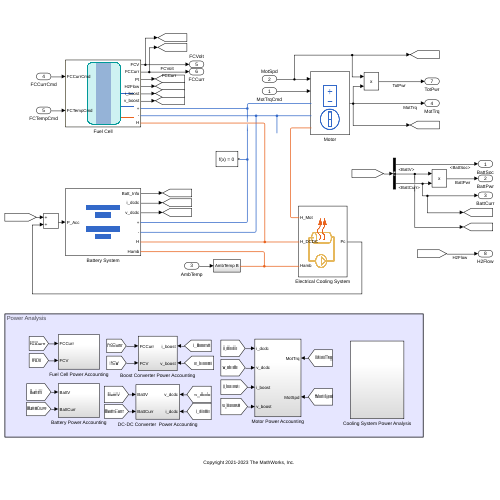
[thumbnail: Simulink's stored preview of the top-level diagram]
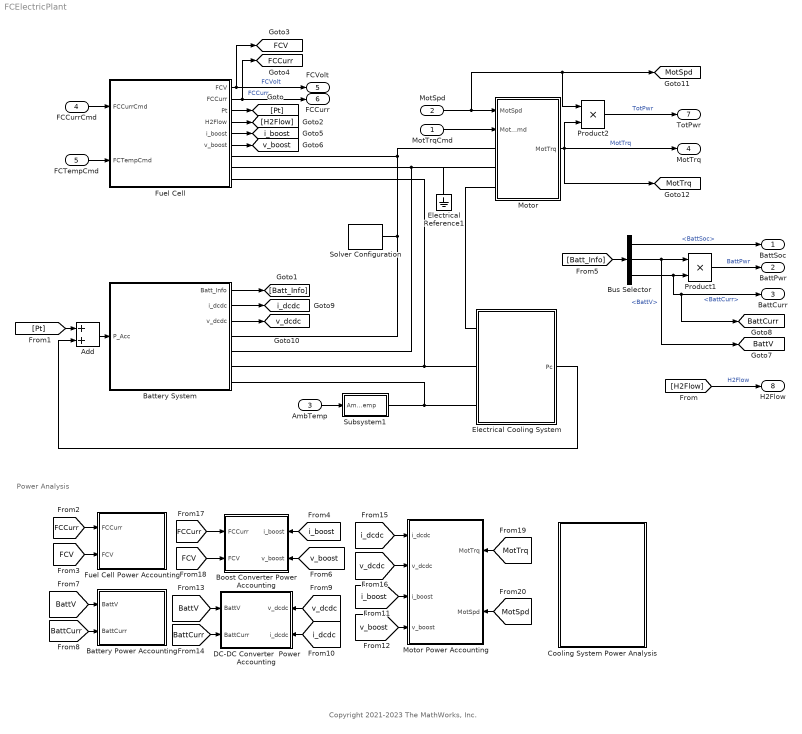
== system FCElectricPlant ==
  note: Power Analysis
  note: Copyright 2021-2023 The MathWorks, Inc.
  MotTrqCmd : Inport
  MotSpd : Inport  Port=2
  AmbTemp : Inport  Port=3
  FCCurrCmd : Inport  Port=4
  FCTempCmd : Inport  Port=5
  Add : Sum
  Battery Power Accounting : Subsystem
  Battery System : Subsystem  VariantControl=0
      mask Display: image('battery_system_IMAGE.png'); % Use "Edit Image" on toolstrip to change.
  Boost Converter Power Accounting : Subsystem
      settings: PortSchema="{\"entries\":[{\"content\":{\"sides\":[{\"content\":{\"connectorIds\":[\"In1\",\"In2\"]},\"type\":\"ConnectorPlacement.EquallySpacedRectSide\",\"uuid\":\"d2a551ba-eb44-482a-8b60-e976053edff0\"},{\"content\":{\"connectorIds\":[\"In3\",\"In4\"],\"side\":\"RIGHT\"},\"type\":\"ConnectorPlacement.EquallySpacedRectSide\",\"uuid\":\"1d9e63ac-fab3-49c5-b28c-f2426adc8d48\"},{\"content\":{\"connectorIds\":[],\"side\":\"TOP\"},\"type\":\"ConnectorPlacement.EquallySpacedRectSide\",\"uuid\":\"1e6d9942-601c-4fdd-92d2-eb031f598739\"}]},\"type\":\"ConnectorPlacement.EquallySpacedConnector\",\"uuid\":\"1b61a22e-efb0-44fb-b76b-176eebc7031d\"}],\"packageUris\":[\"http://schema.mathworks.com/mf0/Connector/R2020b\"],\"version\":\"1.0\"}"
  Bus Selector : BusSelector  OutputSignals=BattSoc,BattV,BattCurr
  Cooling System Power Analysis : Subsystem
  DC-DC Converter  Power Accounting : Subsystem
      settings: PortSchema="{\"entries\":[{\"content\":{\"sides\":[{\"content\":{\"connectorIds\":[\"In1\",\"In2\"]},\"type\":\"ConnectorPlacement.EquallySpacedRectSide\",\"uuid\":\"d2a551ba-eb44-482a-8b60-e976053edff0\"},{\"content\":{\"connectorIds\":[\"In3\",\"In4\"],\"side\":\"RIGHT\"},\"type\":\"ConnectorPlacement.EquallySpacedRectSide\",\"uuid\":\"1d9e63ac-fab3-49c5-b28c-f2426adc8d48\"},{\"content\":{\"connectorIds\":[],\"side\":\"TOP\"},\"type\":\"ConnectorPlacement.EquallySpacedRectSide\",\"uuid\":\"1e6d9942-601c-4fdd-92d2-eb031f598739\"}]},\"type\":\"ConnectorPlacement.EquallySpacedConnector\",\"uuid\":\"1b61a22e-efb0-44fb-b76b-176eebc7031d\"}],\"packageUris\":[\"http://schema.mathworks.com/mf0/Connector/R2020b\"],\"version\":\"1.0\"}"
  Electrical Cooling System : Subsystem
      mask Display: image('cooling_active1loop_IMAGE.png'); % Use "Edit Image" on toolstrip to change.
  Electrical Reference1 : fl_lib/Electrical/Electrical Elements/Electrical Reference
  Fuel Cell : Subsystem  VariantControl=0
      mask Display: image('fuel_cell_converter_IMAGE.png'); % Use "Edit Image" on toolstrip to change.
  Fuel Cell Power Accounting : Subsystem
  Motor : Subsystem
      mask Display: image('emotor_simplified_IMAGE.png'); % Use "Edit Image" on toolstrip to change.
  Motor Power Accounting : Subsystem
      settings: PortSchema="{\"entries\":[{\"content\":{\"sides\":[{\"content\":{\"connectorIds\":[\"In1\",\"In2\",\"In3\",\"In4\"]},\"type\":\"ConnectorPlacement.EquallySpacedRectSide\",\"uuid\":\"6ec4812d-f6a8-428e-ab71-0e64a82e557b\"},{\"content\":{\"connectorIds\":[\"In5\",\"In6\"],\"side\":\"RIGHT\"},\"type\":\"ConnectorPlacement.EquallySpacedRectSide\",\"uuid\":\"a1192fa4-ef5f-453a-86cc-222a9b7953b2\"},{\"content\":{\"connectorIds\":[],\"side\":\"TOP\"},\"type\":\"ConnectorPlacement.EquallySpacedRectSide\",\"uuid\":\"391d63f3-8abc-4151-8569-a2196654f909\"}]},\"type\":\"ConnectorPlacement.EquallySpacedConnector\",\"uuid\":\"660d9ac6-f464-40a8-9602-452be741244a\"}],\"packageUris\":[\"http://schema.mathworks.com/mf0/Connector/R2020b\"],\"version\":\"1.0\"}"
  Product1 : Product
  Product2 : Product
  Solver Configuration : nesl_utility/Solver Configuration  PhysicalDomain=network_engine_domain  SubClassName=solver  LeftPortType=input  RightPortType=generic  Tones=[]  Harmonics=[]  SimulateNoise=off  Profile=off  UseLocalSampling=off  EnableSwitchedLinearOptims=on  FrequencyDomain=off  UseCCode=off  RelTol=0.001  AbsTol=1e-06  MinStep=1e-09  ToWorkspace=off  RevertToSquareIcSolve=off  NumHomotopyIterations=100  PhasorMode=off  PhasorModeNumHarmonics=1  ConsistencySolver=NEWTON_FTOL  IndexReductionMethod=DerivativeReplacement  DoDC=off  ResidualTolerance=1e-09  ConsistencyTolSource=GLOBAL  ConsistencyAbsTol=0.001  ConsistencyRelTol=0.001  ConsistencyTolFactor=0.001  UseLocalSolver=off  LocalSolverChoice=NE_BACKWARD_EULER_ADVANCER  ResolveIndetEquations=on  FunctionEvalNumThread=1  LocalSolverSampleTime=1  DoFixedCost=off  MaxNonlinIter=3  MaxModeIter=2  ComputeImpulses=on  ImpulseIterations=2  LinearAlgebra=Sparse  LinearAlgebraNumThread=0  EquationFormulation=NE_TIME_EF  DelaysMemoryBudget=1024  AutomaticFiltering=off  FilteringTimeConstant=0.001  PartitionStorageMethod=AS_NEEDED  PartitionMemoryBudget=1024  PartitionMethod=FAST  MultibodyUseLocalSolver=off  MultibodyLocalSolverChoice=ODE1  MultibodyLocalSolverSampleTime=0.001
  Subsystem1 : Subsystem
  BattSoc : Outport  VectorParamsAs1DForOutWhenUnconnected=off
  BattPwr : Outport  Port=2  VectorParamsAs1DForOutWhenUnconnected=off
  BattCurr : Outport  Port=3  VectorParamsAs1DForOutWhenUnconnected=off
  MotTrq : Outport  Port=4  VectorParamsAs1DForOutWhenUnconnected=off
  FCVolt : Outport  Port=5  VectorParamsAs1DForOutWhenUnconnected=off
  FCCurr : Outport  Port=6  VectorParamsAs1DForOutWhenUnconnected=off
  TotPwr : Outport  Port=7
  H2Flow : Outport  Port=8  VectorParamsAs1DForOutWhenUnconnected=off
  tag scope: BattCurr=global, BattV=global, FCCurr=global, FCV=global, MotSpd=global, MotTrq=global, i_boost=global, i_dcdc=global, v_boost=global, v_dcdc=global
  wires:
  FCTempCmd/1 -> Fuel Cell/2(FCTempCmd)
  Product1/1 -> BattPwr/1  "BattPwr"
  Bus Selector/2 -> Product1/1, [BattV]  "<BattV>"
  AmbTemp/1 -> Subsystem1/1(AmbTemp)
  Bus Selector/1 -> BattSoc/1  "<BattSoc>"
  Motor/1(MotTrq) -> [MotTrq], Product2/2, MotTrq/1  "MotTrq"
  MotTrqCmd/1 -> Motor/2(MotTrqCmd)
  Bus Selector/3 -> [BattCurr], BattCurr/1, Product1/2  "<BattCurr>"
  FCCurrCmd/1 -> Fuel Cell/1(FCCurrCmd)
  MotSpd/1 -> Product2/1, [MotSpd], Motor/1(MotSpd)
  Fuel Cell/3(Pt) -> [Pt]
  Fuel Cell/1(FCV) -> FCVolt/1, [FCV]  "FCVolt"
  Fuel Cell/2(FCCurr) -> FCCurr/1, [FCCurr]  "FCCurr"
  Battery System/1(Batt_Info) -> [Batt_Info]
  [Batt_Info] -> Bus Selector/1
  Add/1 -> Battery System/1(P_Acc)
  [Pt] -> Add/1
  Electrical Cooling System/1(Pc) -> Add/2
  Product2/1 -> TotPwr/1  "TotPwr"
  Fuel Cell/4(H2Flow) -> [H2Flow]
  [H2Flow] -> H2Flow/1  "H2Flow"
  Fuel Cell/5(i_boost) -> [i_boost]
  Fuel Cell/6(v_boost) -> [v_boost]
  Battery System/2(i_dcdc) -> [i_dcdc]
  Battery System/3(v_dcdc) -> [v_dcdc]
  [i_boost] -> Boost Converter Power Accounting/3(i_boost)
  [FCV] -> Fuel Cell Power Accounting/2(FCV)
  [FCV] -> Boost Converter Power Accounting/2(FCV)
  [FCCurr] -> Boost Converter Power Accounting/1(FCCurr)
  [FCCurr] -> Fuel Cell Power Accounting/1(FCCurr)
  [v_boost] -> Boost Converter Power Accounting/4(v_boost)
  [BattV] -> DC-DC Converter  Power Accounting/1(BattV)
  [i_dcdc] -> DC-DC Converter  Power Accounting/4(i_dcdc)
  [BattV] -> Battery Power Accounting/1(BattV)
  [v_dcdc] -> DC-DC Converter  Power Accounting/3(v_dcdc)
  [BattCurr] -> Battery Power Accounting/2(BattCurr)
  [BattCurr] -> DC-DC Converter  Power Accounting/2(BattCurr)
  [v_dcdc] -> Motor Power Accounting/2(v_dcdc)
  [i_boost] -> Motor Power Accounting/3(i_boost)
  [MotSpd] -> Motor Power Accounting/6(MotSpd)
  [i_dcdc] -> Motor Power Accounting/1(i_dcdc)
  [MotTrq] -> Motor Power Accounting/5(MotTrq)
  [v_boost] -> Motor Power Accounting/4(v_boost)
  connections:
  Battery System/RConn2 -- Electrical Reference1/LConn1 -- Motor/LConn2 -- Fuel Cell/RConn2
  Battery System/RConn1 -- Solver Configuration/RConn1 -- Motor/LConn1 -- Fuel Cell/RConn1
  Electrical Cooling System/LConn2 -- Fuel Cell/RConn3 -- Battery System/RConn3
  Electrical Cooling System/LConn1 -- Motor/LConn3
  Electrical Cooling System/LConn3 -- Battery System/RConn4 -- Subsystem1/RConn1
